simulink model "MdXX_RspToNetWork"  (R2024b)
settings: Solver=FixedStepDiscrete  StartTime=0.0  StopTime=10.0  FixedStep=0.01  RelTol=1e-3
(part 1 of 3)
settings Model: Creator=sn2xws  LastModifiedBy=sn55gm
settings Model: ModifiedHistory=|
  | 2024.8.20 v3.0.0 557增加Md53 Md56
  | 2024.10.15 V3.0.1 新增Md57 Md58
  | 25.7.8 V3.13.0 新增Md61 Md62
settings SolverCC: AlgebraicLoopSolver=TrustRegion
settings DataIOCC: SaveFormat=StructureWithTime  ReturnWorkspaceOutputs=off
settings OptimizationCC: DefaultParameterBehavior=Inlined  EnhancedBackFolding=on  PassReuseOutputArgsAs=Individual arguments  ZeroExternalMemoryAtStartup=off  ZeroInternalMemoryAtStartup=off  OptimizeBlockOrder=speed  DifferentSizesBufferReuse=on  OptimizationCustomize=off  EfficientTunableParamExpr=on
settings DebuggingCC: ParameterTunabilityLossMsg=error  UnconnectedInputMsg=warning  UnconnectedOutputMsg=warning  UnconnectedLineMsg=warning  ArithmeticOperatorsInVariantConditions=warning
settings ModelReferenceCC: EnableRefExpFcnMdlSchedulingChecks=on  ModelReferenceNumInstancesAllowed=Single
settings SFSimCC: MATLABDynamicMemAlloc=off  CustomCodeUndefinedFunction=UseInterfaceOnly
settings RTWCC: Description=AUTOSAR  SystemTargetFile=autosar.tlc  GenCodeOnly=on  TemplateMakefile=ert_default_tmf  GenerateReport=on  IncludeHyperlinkInReport=on  LaunchReport=on  DataTypeReplacement=CDataTypesFixedWidth  GenerateTraceInfo=on  GenerateTraceReport=on  GenerateTraceReportSl=on  GenerateTraceReportSf=on  GenerateTraceReportEml=on  GenerateCodeMetricsReport=on  GPUComputeCapability=3.5
settings CodeAppCC: ForceParamTrailComments=on  IgnoreCustomStorageClasses=off  OperatorAnnotations=on  SimulinkDataObjDesc=on  SFDataObjDesc=on  InsertBlockDesc=on
settings STFCustomTargetCC: TargetLangStandard=C99 (ISO)  MultiwordLength=256  ParMdlRefBuildCompliant=on  CompOptLevelCompliant=on  IncludeMdlTerminateFcn=off  CombineOutputUpdateFcns=on  SuppressErrorStatus=on  ERTCustomFileBanners=on  SupportNonFinite=off  SupportComplex=off  SupportContinuousTime=off  SupportNonInlinedSFcns=off  RemoveResetFunc=on  MATLABClassNameForMDSCustomization=Simulink.SoftwareTarget.ERTCustomization  AutosarCompliant=on  UseToolchainInfoCompliant=on  LookupTableObjectStructAxisOrder=2,1,3,4,...  LUTObjectStructOrderEvenSpacing=Size,Table,Breakpoints  SystemTargetFile=autosar.tlc
settings ERTTargetCC: TargetLangStandard=C99 (ISO)  ConcurrentExecutionCompliant=off  IncludeMdlTerminateFcn=off  SuppressErrorStatus=on  SupportNonFinite=off  SupportComplex=off  ModelStepFunctionPrototypeControlCompliant=off  CPPClassGenCompliant=off  AutosarCompliant=on  LookupTableObjectStructAxisOrder=2,1,3,4,...  LUTObjectStructOrderEvenSpacing=Size,Table,Breakpoints  ERTCustomFileTemplate=example_file_process.tlc  ERTFilePackagingFormat=Compact  BooleanTrueId=TRUE  BooleanFalseId=FALSE  DynamicArrayContainerType=coder::array

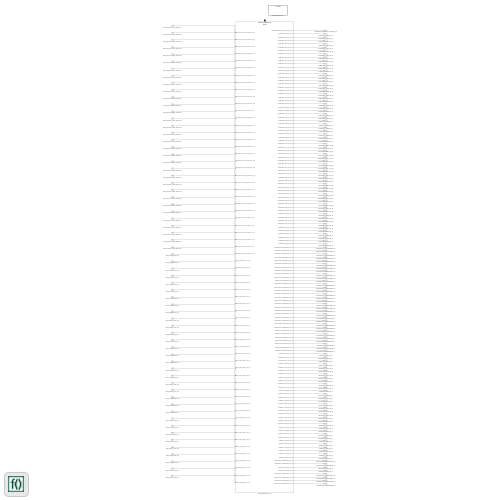
[thumbnail: Simulink's stored preview of the top-level diagram]
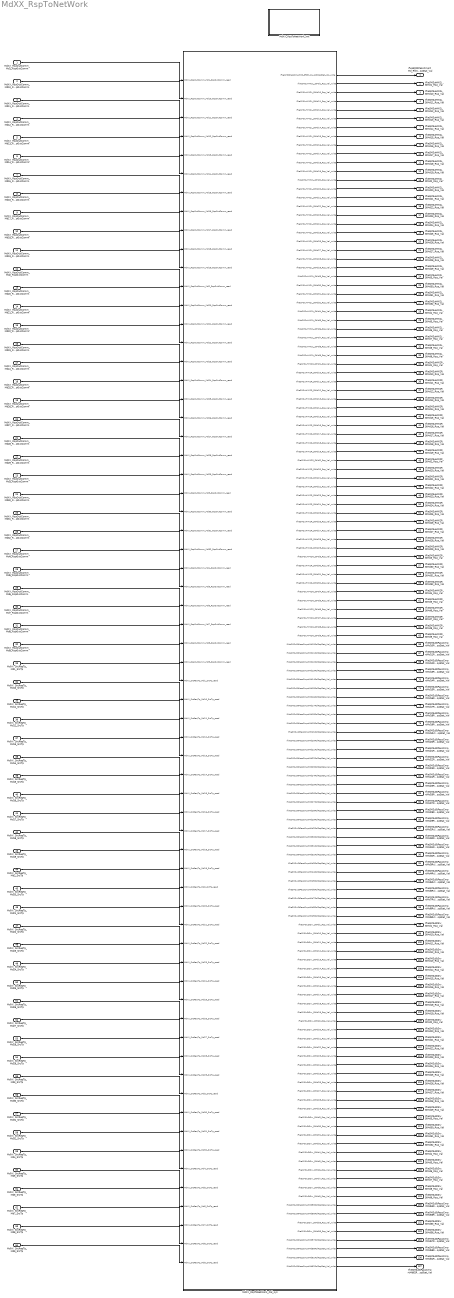
== system MdXX_RspToNetWork ==
  MdXX_RspOutComm_Md1_RspOutComm : Inport  OutDataTypeStr=uint8  PortDimensions=1
  MdXX_RspOutComm_Md10_RspOutComm : Inport  Port=2  OutDataTypeStr=uint8  PortDimensions=1
  MdXX_RspOutComm_Md11_RspOutComm : Inport  Port=3  OutDataTypeStr=uint8  PortDimensions=1
  MdXX_RspOutComm_Md12_RspOutComm : Inport  Port=4  OutDataTypeStr=uint8  PortDimensions=1
  MdXX_RspOutComm_Md13_RspOutComm : Inport  Port=5  OutDataTypeStr=uint8  PortDimensions=1
  MdXX_RspOutComm_Md14_RspOutComm : Inport  Port=6  OutDataTypeStr=uint8  PortDimensions=1
  MdXX_RspOutComm_Md15_RspOutComm : Inport  Port=7  OutDataTypeStr=uint8  PortDimensions=1
  MdXX_RspOutComm_Md16_RspOutComm : Inport  Port=8  OutDataTypeStr=uint8  PortDimensions=1
  MdXX_RspOutComm_Md17_RspOutComm : Inport  Port=9  OutDataTypeStr=uint8  PortDimensions=1
  MdXX_RspOutComm_Md18_RspOutComm : Inport  Port=10  OutDataTypeStr=uint8  PortDimensions=1
  MdXX_RspOutComm_Md19_RspOutComm : Inport  Port=11  OutDataTypeStr=uint8  PortDimensions=1
  MdXX_RspOutComm_Md2_RspOutComm : Inport  Port=12  OutDataTypeStr=uint8  PortDimensions=1
  MdXX_RspOutComm_Md20_RspOutComm : Inport  Port=13  OutDataTypeStr=uint8  PortDimensions=1
  MdXX_RspOutComm_Md21_RspOutComm : Inport  Port=14  OutDataTypeStr=uint8  PortDimensions=1
  MdXX_RspOutComm_Md22_RspOutComm : Inport  Port=15  OutDataTypeStr=uint8  PortDimensions=1
  MdXX_RspOutComm_Md23_RspOutComm : Inport  Port=16  OutDataTypeStr=uint8  PortDimensions=1
  MdXX_RspOutComm_Md24_RspOutComm : Inport  Port=17  OutDataTypeStr=uint8  PortDimensions=1
  MdXX_RspOutComm_Md25_RspOutComm : Inport  Port=18  OutDataTypeStr=uint8  PortDimensions=1
  MdXX_RspOutComm_Md26_RspOutComm : Inport  Port=19  OutDataTypeStr=uint8  PortDimensions=1
  MdXX_RspOutComm_Md27_RspOutComm : Inport  Port=20  OutDataTypeStr=uint8  PortDimensions=1
  MdXX_RspOutComm_Md28_RspOutComm : Inport  Port=21  OutDataTypeStr=uint8  PortDimensions=1
  MdXX_RspOutComm_Md29_RspOutComm : Inport  Port=22  OutDataTypeStr=uint8  PortDimensions=1
  MdXX_RspOutComm_Md3_RspOutComm : Inport  Port=23  OutDataTypeStr=uint8  PortDimensions=1
  MdXX_RspOutComm_Md30_RspOutComm : Inport  Port=24  OutDataTypeStr=uint8  PortDimensions=1
  MdXX_RspOutComm_Md31_RspOutComm : Inport  Port=25  OutDataTypeStr=uint8  PortDimensions=1
  MdXX_RspOutComm_Md32_RspOutComm : Inport  Port=26  OutDataTypeStr=uint8  PortDimensions=1
  MdXX_RspOutComm_Md4_RspOutComm : Inport  Port=27  OutDataTypeStr=uint8  PortDimensions=1
  MdXX_RspOutComm_Md5_RspOutComm : Inport  Port=28  OutDataTypeStr=uint8  PortDimensions=1
  MdXX_RspOutComm_Md6_RspOutComm : Inport  Port=29  OutDataTypeStr=uint8  PortDimensions=1
  MdXX_RspOutComm_Md7_RspOutComm : Inport  Port=30  OutDataTypeStr=uint8  PortDimensions=1
  MdXX_RspOutComm_Md8_RspOutComm : Inport  Port=31  OutDataTypeStr=uint8  PortDimensions=1
  MdXX_RspOutComm_Md9_RspOutComm : Inport  Port=32  OutDataTypeStr=uint8  PortDimensions=1
  MdXX_SrcReqTp_Md1_SrcTp : Inport  Port=33  OutDataTypeStr=Enum: SrcReqTp1  PortDimensions=1
  MdXX_SrcReqTp_Md10_SrcTp : Inport  Port=34  OutDataTypeStr=Enum: SrcReqTp1  PortDimensions=1
  MdXX_SrcReqTp_Md11_SrcTp : Inport  Port=35  OutDataTypeStr=Enum: SrcReqTp1  PortDimensions=1
  MdXX_SrcReqTp_Md12_SrcTp : Inport  Port=36  OutDataTypeStr=Enum: SrcReqTp1  PortDimensions=1
  MdXX_SrcReqTp_Md13_SrcTp : Inport  Port=37  OutDataTypeStr=Enum: SrcReqTp1  PortDimensions=1
  MdXX_SrcReqTp_Md14_SrcTp : Inport  Port=38  OutDataTypeStr=Enum: SrcReqTp1  PortDimensions=1
  MdXX_SrcReqTp_Md15_SrcTp : Inport  Port=39  OutDataTypeStr=Enum: SrcReqTp1  PortDimensions=1
  MdXX_SrcReqTp_Md16_SrcTp : Inport  Port=40  OutDataTypeStr=Enum: SrcReqTp1  PortDimensions=1
  MdXX_SrcReqTp_Md17_SrcTp : Inport  Port=41  OutDataTypeStr=Enum: SrcReqTp1  PortDimensions=1
  MdXX_SrcReqTp_Md18_SrcTp : Inport  Port=42  OutDataTypeStr=Enum: SrcReqTp1  PortDimensions=1
  MdXX_SrcReqTp_Md19_SrcTp : Inport  Port=43  OutDataTypeStr=Enum: SrcReqTp1  PortDimensions=1
  MdXX_SrcReqTp_Md2_SrcTp : Inport  Port=44  OutDataTypeStr=Enum: SrcReqTp1  PortDimensions=1
  MdXX_SrcReqTp_Md20_SrcTp : Inport  Port=45  OutDataTypeStr=Enum: SrcReqTp1  PortDimensions=1
  MdXX_SrcReqTp_Md21_SrcTp : Inport  Port=46  OutDataTypeStr=Enum: SrcReqTp1  PortDimensions=1
  MdXX_SrcReqTp_Md22_SrcTp : Inport  Port=47  OutDataTypeStr=Enum: SrcReqTp1  PortDimensions=1
  MdXX_SrcReqTp_Md23_SrcTp : Inport  Port=48  OutDataTypeStr=Enum: SrcReqTp1  PortDimensions=1
  MdXX_SrcReqTp_Md24_SrcTp : Inport  Port=49  OutDataTypeStr=Enum: SrcReqTp1  PortDimensions=1
  MdXX_SrcReqTp_Md25_SrcTp : Inport  Port=50  OutDataTypeStr=Enum: SrcReqTp1  PortDimensions=1
  MdXX_SrcReqTp_Md26_SrcTp : Inport  Port=51  OutDataTypeStr=Enum: SrcReqTp1  PortDimensions=1
  MdXX_SrcReqTp_Md27_SrcTp : Inport  Port=52  OutDataTypeStr=Enum: SrcReqTp1  PortDimensions=1
  MdXX_SrcReqTp_Md28_SrcTp : Inport  Port=53  OutDataTypeStr=Enum: SrcReqTp1  PortDimensions=1
  MdXX_SrcReqTp_Md29_SrcTp : Inport  Port=54  OutDataTypeStr=Enum: SrcReqTp1  PortDimensions=1
  MdXX_SrcReqTp_Md3_SrcTp : Inport  Port=55  OutDataTypeStr=Enum: SrcReqTp1  PortDimensions=1
  MdXX_SrcReqTp_Md30_SrcTp : Inport  Port=56  OutDataTypeStr=Enum: SrcReqTp1  PortDimensions=1
  MdXX_SrcReqTp_Md31_SrcTp : Inport  Port=57  OutDataTypeStr=Enum: SrcReqTp1  PortDimensions=1
  MdXX_SrcReqTp_Md32_SrcTp : Inport  Port=58  OutDataTypeStr=Enum: SrcReqTp1  PortDimensions=1
  MdXX_SrcReqTp_Md4_SrcTp : Inport  Port=59  OutDataTypeStr=Enum: SrcReqTp1  PortDimensions=1
  MdXX_SrcReqTp_Md5_SrcTp : Inport  Port=60  OutDataTypeStr=Enum: SrcReqTp1  PortDimensions=1
  MdXX_SrcReqTp_Md6_SrcTp : Inport  Port=61  OutDataTypeStr=Enum: SrcReqTp1  PortDimensions=1
  MdXX_SrcReqTp_Md7_SrcTp : Inport  Port=62  OutDataTypeStr=Enum: SrcReqTp1  PortDimensions=1
  MdXX_SrcReqTp_Md8_SrcTp : Inport  Port=63  OutDataTypeStr=Enum: SrcReqTp1  PortDimensions=1
  MdXX_SrcReqTp_Md9_SrcTp : Inport  Port=64  OutDataTypeStr=Enum: SrcReqTp1  PortDimensions=1
  MdXX_RspToNetWork_Cal_sys : Subsystem
  MdXX_RspToNetWork_Init : Subsystem
  IfVeSMStPassCmprtMd_RfCtrl_Sw_RclRspStat_Val : Outport  OutDataTypeStr=uint8  PortDimensions=1  VectorParamsAs1DForOutWhenUnconnected=off
  IfVeSMSuHMI2L_StMd1_Rsp_Val : Outport  Port=2  OutDataTypeStr=uint8  PortDimensions=1  VectorParamsAs1DForOutWhenUnconnected=off
  IfVeSMSuHMI2L_StMd10_Rsp_Val : Outport  Port=3  OutDataTypeStr=uint8  PortDimensions=1  VectorParamsAs1DForOutWhenUnconnected=off
  IfVeSMSuHMI2L_StMd11_Rsp_Val : Outport  Port=4  OutDataTypeStr=uint8  PortDimensions=1  VectorParamsAs1DForOutWhenUnconnected=off
  IfVeSMSuHMI2L_StMd12_Rsp_Val : Outport  Port=5  OutDataTypeStr=uint8  PortDimensions=1  VectorParamsAs1DForOutWhenUnconnected=off
  IfVeSMSuHMI2L_StMd13_Rsp_Val : Outport  Port=6  OutDataTypeStr=uint8  PortDimensions=1  VectorParamsAs1DForOutWhenUnconnected=off
  IfVeSMSuHMI2L_StMd14_Rsp_Val : Outport  Port=7  OutDataTypeStr=uint8  PortDimensions=1  VectorParamsAs1DForOutWhenUnconnected=off
  IfVeSMSuHMI2L_StMd15_Rsp_Val : Outport  Port=8  OutDataTypeStr=uint8  PortDimensions=1  VectorParamsAs1DForOutWhenUnconnected=off
  IfVeSMSuHMI2L_StMd16_Rsp_Val : Outport  Port=9  OutDataTypeStr=uint8  PortDimensions=1  VectorParamsAs1DForOutWhenUnconnected=off
  IfVeSMSuHMI2L_StMd17_Rsp_Val : Outport  Port=10  OutDataTypeStr=uint8  PortDimensions=1  VectorParamsAs1DForOutWhenUnconnected=off
  IfVeSMSuHMI2L_StMd18_Rsp_Val : Outport  Port=11  OutDataTypeStr=uint8  PortDimensions=1  VectorParamsAs1DForOutWhenUnconnected=off
  IfVeSMSuHMI2L_StMd19_Rsp_Val : Outport  Port=12  OutDataTypeStr=uint8  PortDimensions=1  VectorParamsAs1DForOutWhenUnconnected=off
  IfVeSMSuHMI2L_StMd2_Rsp_Val : Outport  Port=13  OutDataTypeStr=uint8  PortDimensions=1  VectorParamsAs1DForOutWhenUnconnected=off
  IfVeSMSuHMI2L_StMd20_Rsp_Val : Outport  Port=14  OutDataTypeStr=uint8  PortDimensions=1  VectorParamsAs1DForOutWhenUnconnected=off
  IfVeSMSuHMI2L_StMd21_Rsp_Val : Outport  Port=15  OutDataTypeStr=uint8  PortDimensions=1  VectorParamsAs1DForOutWhenUnconnected=off
  IfVeSMSuHMI2L_StMd22_Rsp_Val : Outport  Port=16  OutDataTypeStr=uint8  PortDimensions=1  VectorParamsAs1DForOutWhenUnconnected=off
  IfVeSMSuHMI2L_StMd23_Rsp_Val : Outport  Port=17  OutDataTypeStr=uint8  PortDimensions=1  VectorParamsAs1DForOutWhenUnconnected=off
  IfVeSMSuHMI2L_StMd24_Rsp_Val : Outport  Port=18  OutDataTypeStr=uint8  PortDimensions=1  VectorParamsAs1DForOutWhenUnconnected=off
  IfVeSMSuHMI2L_StMd25_Rsp_Val : Outport  Port=19  OutDataTypeStr=uint8  PortDimensions=1  VectorParamsAs1DForOutWhenUnconnected=off
  IfVeSMSuHMI2L_StMd26_Rsp_Val : Outport  Port=20  OutDataTypeStr=uint8  PortDimensions=1  VectorParamsAs1DForOutWhenUnconnected=off
  IfVeSMSuHMI2L_StMd27_Rsp_Val : Outport  Port=21  OutDataTypeStr=uint8  PortDimensions=1  VectorParamsAs1DForOutWhenUnconnected=off
  IfVeSMSuHMI2L_StMd28_Rsp_Val : Outport  Port=22  OutDataTypeStr=uint8  PortDimensions=1  VectorParamsAs1DForOutWhenUnconnected=off
  IfVeSMSuHMI2L_StMd29_Rsp_Val : Outport  Port=23  OutDataTypeStr=uint8  PortDimensions=1  VectorParamsAs1DForOutWhenUnconnected=off
  IfVeSMSuHMI2L_StMd3_Rsp_Val : Outport  Port=24  OutDataTypeStr=uint8  PortDimensions=1  VectorParamsAs1DForOutWhenUnconnected=off
  IfVeSMSuHMI2L_StMd30_Rsp_Val : Outport  Port=25  OutDataTypeStr=uint8  PortDimensions=1  VectorParamsAs1DForOutWhenUnconnected=off
  IfVeSMSuHMI2L_StMd31_Rsp_Val : Outport  Port=26  OutDataTypeStr=uint8  PortDimensions=1  VectorParamsAs1DForOutWhenUnconnected=off
  IfVeSMSuHMI2L_StMd32_Rsp_Val : Outport  Port=27  OutDataTypeStr=uint8  PortDimensions=1  VectorParamsAs1DForOutWhenUnconnected=off
  IfVeSMSuHMI2L_StMd4_Rsp_Val : Outport  Port=28  OutDataTypeStr=uint8  PortDimensions=1  VectorParamsAs1DForOutWhenUnconnected=off
  IfVeSMSuHMI2L_StMd5_Rsp_Val : Outport  Port=29  OutDataTypeStr=uint8  PortDimensions=1  VectorParamsAs1DForOutWhenUnconnected=off
  IfVeSMSuHMI2L_StMd6_Rsp_Val : Outport  Port=30  OutDataTypeStr=uint8  PortDimensions=1  VectorParamsAs1DForOutWhenUnconnected=off
  IfVeSMSuHMI2L_StMd7_Rsp_Val : Outport  Port=31  OutDataTypeStr=uint8  PortDimensions=1  VectorParamsAs1DForOutWhenUnconnected=off
  IfVeSMSuHMI2L_StMd8_Rsp_Val : Outport  Port=32  OutDataTypeStr=uint8  PortDimensions=1  VectorParamsAs1DForOutWhenUnconnected=off
  IfVeSMSuHMI2L_StMd9_Rsp_Val : Outport  Port=33  OutDataTypeStr=uint8  PortDimensions=1  VectorParamsAs1DForOutWhenUnconnected=off
  IfVeSMSuHMI2R_StMd1_Rsp_Val : Outport  Port=34  OutDataTypeStr=uint8  PortDimensions=1  VectorParamsAs1DForOutWhenUnconnected=off
  IfVeSMSuHMI2R_StMd10_Rsp_Val : Outport  Port=35  OutDataTypeStr=uint8  PortDimensions=1  VectorParamsAs1DForOutWhenUnconnected=off
  IfVeSMSuHMI2R_StMd11_Rsp_Val : Outport  Port=36  OutDataTypeStr=uint8  PortDimensions=1  VectorParamsAs1DForOutWhenUnconnected=off
  IfVeSMSuHMI2R_StMd12_Rsp_Val : Outport  Port=37  OutDataTypeStr=uint8  PortDimensions=1  VectorParamsAs1DForOutWhenUnconnected=off
  IfVeSMSuHMI2R_StMd13_Rsp_Val : Outport  Port=38  OutDataTypeStr=uint8  PortDimensions=1  VectorParamsAs1DForOutWhenUnconnected=off
  IfVeSMSuHMI2R_StMd14_Rsp_Val : Outport  Port=39  OutDataTypeStr=uint8  PortDimensions=1  VectorParamsAs1DForOutWhenUnconnected=off
  IfVeSMSuHMI2R_StMd15_Rsp_Val : Outport  Port=40  OutDataTypeStr=uint8  PortDimensions=1  VectorParamsAs1DForOutWhenUnconnected=off
  IfVeSMSuHMI2R_StMd16_Rsp_Val : Outport  Port=41  OutDataTypeStr=uint8  PortDimensions=1  VectorParamsAs1DForOutWhenUnconnected=off
  IfVeSMSuHMI2R_StMd17_Rsp_Val : Outport  Port=42  OutDataTypeStr=uint8  PortDimensions=1  VectorParamsAs1DForOutWhenUnconnected=off
  IfVeSMSuHMI2R_StMd18_Rsp_Val : Outport  Port=43  OutDataTypeStr=uint8  PortDimensions=1  VectorParamsAs1DForOutWhenUnconnected=off
  IfVeSMSuHMI2R_StMd19_Rsp_Val : Outport  Port=44  OutDataTypeStr=uint8  PortDimensions=1  VectorParamsAs1DForOutWhenUnconnected=off
  IfVeSMSuHMI2R_StMd2_Rsp_Val : Outport  Port=45  OutDataTypeStr=uint8  PortDimensions=1  VectorParamsAs1DForOutWhenUnconnected=off
  IfVeSMSuHMI2R_StMd20_Rsp_Val : Outport  Port=46  OutDataTypeStr=uint8  PortDimensions=1  VectorParamsAs1DForOutWhenUnconnected=off
  IfVeSMSuHMI2R_StMd21_Rsp_Val : Outport  Port=47  OutDataTypeStr=uint8  PortDimensions=1  VectorParamsAs1DForOutWhenUnconnected=off
  IfVeSMSuHMI2R_StMd22_Rsp_Val : Outport  Port=48  OutDataTypeStr=uint8  PortDimensions=1  VectorParamsAs1DForOutWhenUnconnected=off
  IfVeSMSuHMI2R_StMd23_Rsp_Val : Outport  Port=49  OutDataTypeStr=uint8  PortDimensions=1  VectorParamsAs1DForOutWhenUnconnected=off
  IfVeSMSuHMI2R_StMd24_Rsp_Val : Outport  Port=50  OutDataTypeStr=uint8  PortDimensions=1  VectorParamsAs1DForOutWhenUnconnected=off
  IfVeSMSuHMI2R_StMd25_Rsp_Val : Outport  Port=51  OutDataTypeStr=uint8  PortDimensions=1  VectorParamsAs1DForOutWhenUnconnected=off
  IfVeSMSuHMI2R_StMd26_Rsp_Val : Outport  Port=52  OutDataTypeStr=uint8  PortDimensions=1  VectorParamsAs1DForOutWhenUnconnected=off
  IfVeSMSuHMI2R_StMd27_Rsp_Val : Outport  Port=53  OutDataTypeStr=uint8  PortDimensions=1  VectorParamsAs1DForOutWhenUnconnected=off
  IfVeSMSuHMI2R_StMd28_Rsp_Val : Outport  Port=54  OutDataTypeStr=uint8  PortDimensions=1  VectorParamsAs1DForOutWhenUnconnected=off
  IfVeSMSuHMI2R_StMd29_Rsp_Val : Outport  Port=55  OutDataTypeStr=uint8  PortDimensions=1  VectorParamsAs1DForOutWhenUnconnected=off
  IfVeSMSuHMI2R_StMd3_Rsp_Val : Outport  Port=56  OutDataTypeStr=uint8  PortDimensions=1  VectorParamsAs1DForOutWhenUnconnected=off
  IfVeSMSuHMI2R_StMd30_Rsp_Val : Outport  Port=57  OutDataTypeStr=uint8  PortDimensions=1  VectorParamsAs1DForOutWhenUnconnected=off
  IfVeSMSuHMI2R_StMd31_Rsp_Val : Outport  Port=58  OutDataTypeStr=uint8  PortDimensions=1  VectorParamsAs1DForOutWhenUnconnected=off
  IfVeSMSuHMI2R_StMd32_Rsp_Val : Outport  Port=59  OutDataTypeStr=uint8  PortDimensions=1  VectorParamsAs1DForOutWhenUnconnected=off
  IfVeSMSuHMI2R_StMd4_Rsp_Val : Outport  Port=60  OutDataTypeStr=uint8  PortDimensions=1  VectorParamsAs1DForOutWhenUnconnected=off
  IfVeSMSuHMI2R_StMd5_Rsp_Val : Outport  Port=61  OutDataTypeStr=uint8  PortDimensions=1  VectorParamsAs1DForOutWhenUnconnected=off
  IfVeSMSuHMI2R_StMd6_Rsp_Val : Outport  Port=62  OutDataTypeStr=uint8  PortDimensions=1  VectorParamsAs1DForOutWhenUnconnected=off
  IfVeSMSuHMI2R_StMd7_Rsp_Val : Outport  Port=63  OutDataTypeStr=uint8  PortDimensions=1  VectorParamsAs1DForOutWhenUnconnected=off
  IfVeSMSuHMI2R_StMd8_Rsp_Val : Outport  Port=64  OutDataTypeStr=uint8  PortDimensions=1  VectorParamsAs1DForOutWhenUnconnected=off
  IfVeSMSuHMI2R_StMd9_Rsp_Val : Outport  Port=65  OutDataTypeStr=uint8  PortDimensions=1  VectorParamsAs1DForOutWhenUnconnected=off
  IfVeSMSuStPassCmprtMd10RclRspStat_Val : Outport  Port=66  OutDataTypeStr=uint8  PortDimensions=1  VectorParamsAs1DForOutWhenUnconnected=off
  IfVeSMSuStPassCmprtMd11RclRspStat_Val : Outport  Port=67  OutDataTypeStr=uint8  PortDimensions=1  VectorParamsAs1DForOutWhenUnconnected=off
  IfVeSMSuStPassCmprtMd12RclRspStat_Val : Outport  Port=68  OutDataTypeStr=uint8  PortDimensions=1  VectorParamsAs1DForOutWhenUnconnected=off
  IfVeSMSuStPassCmprtMd13RclRspStat_Val : Outport  Port=69  OutDataTypeStr=uint8  PortDimensions=1  VectorParamsAs1DForOutWhenUnconnected=off
  IfVeSMSuStPassCmprtMd14RclRspStat_Val : Outport  Port=70  OutDataTypeStr=uint8  PortDimensions=1  VectorParamsAs1DForOutWhenUnconnected=off
  IfVeSMSuStPassCmprtMd15RclRspStat_Val : Outport  Port=71  OutDataTypeStr=uint8  PortDimensions=1  VectorParamsAs1DForOutWhenUnconnected=off
  IfVeSMSuStPassCmprtMd16RclRspStat_Val : Outport  Port=72  OutDataTypeStr=uint8  PortDimensions=1  VectorParamsAs1DForOutWhenUnconnected=off
  IfVeSMSuStPassCmprtMd17RclRspStat_Val : Outport  Port=73  OutDataTypeStr=uint8  PortDimensions=1  VectorParamsAs1DForOutWhenUnconnected=off
  IfVeSMSuStPassCmprtMd18RclRspStat_Val : Outport  Port=74  OutDataTypeStr=uint8  PortDimensions=1  VectorParamsAs1DForOutWhenUnconnected=off
  IfVeSMSuStPassCmprtMd19RclRspStat_Val : Outport  Port=75  OutDataTypeStr=uint8  PortDimensions=1  VectorParamsAs1DForOutWhenUnconnected=off
  IfVeSMSuStPassCmprtMd1RclRspStat_Val : Outport  Port=76  OutDataTypeStr=uint8  PortDimensions=1  VectorParamsAs1DForOutWhenUnconnected=off
  IfVeSMSuStPassCmprtMd20RclRspStat_Val : Outport  Port=77  OutDataTypeStr=uint8  PortDimensions=1  VectorParamsAs1DForOutWhenUnconnected=off
  IfVeSMSuStPassCmprtMd21RclRspStat_Val : Outport  Port=78  OutDataTypeStr=uint8  PortDimensions=1  VectorParamsAs1DForOutWhenUnconnected=off
  IfVeSMSuStPassCmprtMd22RclRspStat_Val : Outport  Port=79  OutDataTypeStr=uint8  PortDimensions=1  VectorParamsAs1DForOutWhenUnconnected=off
  IfVeSMSuStPassCmprtMd23RclRspStat_Val : Outport  Port=80  OutDataTypeStr=uint8  PortDimensions=1  VectorParamsAs1DForOutWhenUnconnected=off
  IfVeSMSuStPassCmprtMd24RclRspStat_Val : Outport  Port=81  OutDataTypeStr=uint8  PortDimensions=1  VectorParamsAs1DForOutWhenUnconnected=off
  IfVeSMSuStPassCmprtMd25RclRspStat_Val : Outport  Port=82  OutDataTypeStr=uint8  PortDimensions=1  VectorParamsAs1DForOutWhenUnconnected=off
  IfVeSMSuStPassCmprtMd26RclRspStat_Val : Outport  Port=83  OutDataTypeStr=uint8  PortDimensions=1  VectorParamsAs1DForOutWhenUnconnected=off
  IfVeSMSuStPassCmprtMd27RclRspStat_Val : Outport  Port=84  OutDataTypeStr=uint8  PortDimensions=1  VectorParamsAs1DForOutWhenUnconnected=off
  IfVeSMSuStPassCmprtMd28RclRspStat_Val : Outport  Port=85  OutDataTypeStr=uint8  PortDimensions=1  VectorParamsAs1DForOutWhenUnconnected=off
  IfVeSMSuStPassCmprtMd29RclRspStat_Val : Outport  Port=86  OutDataTypeStr=uint8  PortDimensions=1  VectorParamsAs1DForOutWhenUnconnected=off
  IfVeSMSuStPassCmprtMd2RclRspStat_Val : Outport  Port=87  OutDataTypeStr=uint8  PortDimensions=1  VectorParamsAs1DForOutWhenUnconnected=off
  IfVeSMSuStPassCmprtMd30RclRspStat_Val : Outport  Port=88  OutDataTypeStr=uint8  PortDimensions=1  VectorParamsAs1DForOutWhenUnconnected=off
  IfVeSMSuStPassCmprtMd31RclRspStat_Val : Outport  Port=89  OutDataTypeStr=uint8  PortDimensions=1  VectorParamsAs1DForOutWhenUnconnected=off
  IfVeSMSuStPassCmprtMd32RclRspStat_Val : Outport  Port=90  OutDataTypeStr=uint8  PortDimensions=1  VectorParamsAs1DForOutWhenUnconnected=off
  IfVeSMSuStPassCmprtMd3RclRspStat_Val : Outport  Port=91  OutDataTypeStr=uint8  PortDimensions=1  VectorParamsAs1DForOutWhenUnconnected=off
  IfVeSMSuStPassCmprtMd4RclRspStat_Val : Outport  Port=92  OutDataTypeStr=uint8  PortDimensions=1  VectorParamsAs1DForOutWhenUnconnected=off
  IfVeSMSuStPassCmprtMd5RclRspStat_Val : Outport  Port=93  OutDataTypeStr=uint8  PortDimensions=1  VectorParamsAs1DForOutWhenUnconnected=off
  IfVeSMSuStPassCmprtMd6RclRspStat_Val : Outport  Port=94  OutDataTypeStr=uint8  PortDimensions=1  VectorParamsAs1DForOutWhenUnconnected=off
  IfVeSMSuStPassCmprtMd7RclRspStat_Val : Outport  Port=95  OutDataTypeStr=uint8  PortDimensions=1  VectorParamsAs1DForOutWhenUnconnected=off
  IfVeSMSuStPassCmprtMd8RclRspStat_Val : Outport  Port=96  OutDataTypeStr=uint8  PortDimensions=1  VectorParamsAs1DForOutWhenUnconnected=off
  IfVeSMSuStPassCmprtMd9RclRspStat_Val : Outport  Port=97  OutDataTypeStr=uint8  PortDimensions=1  VectorParamsAs1DForOutWhenUnconnected=off
  IfVeSMSuStSrv_StMd1_Rsp_Val : Outport  Port=98  OutDataTypeStr=uint8  PortDimensions=1  VectorParamsAs1DForOutWhenUnconnected=off
  IfVeSMSuStSrv_StMd10_Rsp_Val : Outport  Port=99  OutDataTypeStr=uint8  PortDimensions=1  VectorParamsAs1DForOutWhenUnconnected=off
  IfVeSMSuStSrv_StMd11_Rsp_Val : Outport  Port=100  OutDataTypeStr=uint8  PortDimensions=1  VectorParamsAs1DForOutWhenUnconnected=off
  IfVeSMSuStSrv_StMd12_Rsp_Val : Outport  Port=101  OutDataTypeStr=uint8  PortDimensions=1  VectorParamsAs1DForOutWhenUnconnected=off
  IfVeSMSuStSrv_StMd13_Rsp_Val : Outport  Port=102  OutDataTypeStr=uint8  PortDimensions=1  VectorParamsAs1DForOutWhenUnconnected=off
  IfVeSMSuStSrv_StMd14_Rsp_Val : Outport  Port=103  OutDataTypeStr=uint8  PortDimensions=1  VectorParamsAs1DForOutWhenUnconnected=off
  IfVeSMSuStSrv_StMd15_Rsp_Val : Outport  Port=104  OutDataTypeStr=uint8  PortDimensions=1  VectorParamsAs1DForOutWhenUnconnected=off
  IfVeSMSuStSrv_StMd16_Rsp_Val : Outport  Port=105  OutDataTypeStr=uint8  PortDimensions=1  VectorParamsAs1DForOutWhenUnconnected=off
  IfVeSMSuStSrv_StMd17_Rsp_Val : Outport  Port=106  OutDataTypeStr=uint8  PortDimensions=1  VectorParamsAs1DForOutWhenUnconnected=off
  IfVeSMSuStSrv_StMd18_Rsp_Val : Outport  Port=107  OutDataTypeStr=uint8  PortDimensions=1  VectorParamsAs1DForOutWhenUnconnected=off
  IfVeSMSuStSrv_StMd19_Rsp_Val : Outport  Port=108  OutDataTypeStr=uint8  PortDimensions=1  VectorParamsAs1DForOutWhenUnconnected=off
  IfVeSMSuStSrv_StMd2_Rsp_Val : Outport  Port=109  OutDataTypeStr=uint8  PortDimensions=1  VectorParamsAs1DForOutWhenUnconnected=off
  IfVeSMSuStSrv_StMd20_Rsp_Val : Outport  Port=110  OutDataTypeStr=uint8  PortDimensions=1  VectorParamsAs1DForOutWhenUnconnected=off
  IfVeSMSuStSrv_StMd21_Rsp_Val : Outport  Port=111  OutDataTypeStr=uint8  PortDimensions=1  VectorParamsAs1DForOutWhenUnconnected=off
  IfVeSMSuStSrv_StMd22_Rsp_Val : Outport  Port=112  OutDataTypeStr=uint8  PortDimensions=1  VectorParamsAs1DForOutWhenUnconnected=off
  IfVeSMSuStSrv_StMd23_Rsp_Val : Outport  Port=113  OutDataTypeStr=uint8  PortDimensions=1  VectorParamsAs1DForOutWhenUnconnected=off
  IfVeSMSuStSrv_StMd24_Rsp_Val : Outport  Port=114  OutDataTypeStr=uint8  PortDimensions=1  VectorParamsAs1DForOutWhenUnconnected=off
  IfVeSMSuStSrv_StMd25_Rsp_Val : Outport  Port=115  OutDataTypeStr=uint8  PortDimensions=1  VectorParamsAs1DForOutWhenUnconnected=off
  IfVeSMSuStSrv_StMd26_Rsp_Val : Outport  Port=116  OutDataTypeStr=uint8  PortDimensions=1  VectorParamsAs1DForOutWhenUnconnected=off
  IfVeSMSuStSrv_StMd27_Rsp_Val : Outport  Port=117  OutDataTypeStr=uint8  PortDimensions=1  VectorParamsAs1DForOutWhenUnconnected=off
  IfVeSMSuStSrv_StMd28_Rsp_Val : Outport  Port=118  OutDataTypeStr=uint8  PortDimensions=1  VectorParamsAs1DForOutWhenUnconnected=off
  IfVeSMSuStSrv_StMd29_Rsp_Val : Outport  Port=119  OutDataTypeStr=uint8  PortDimensions=1  VectorParamsAs1DForOutWhenUnconnected=off
  IfVeSMSuStSrv_StMd3_Rsp_Val : Outport  Port=120  OutDataTypeStr=uint8  PortDimensions=1  VectorParamsAs1DForOutWhenUnconnected=off
  IfVeSMSuStSrv_StMd30_Rsp_Val : Outport  Port=121  OutDataTypeStr=uint8  PortDimensions=1  VectorParamsAs1DForOutWhenUnconnected=off
  IfVeSMSuStSrv_StMd31_Rsp_Val : Outport  Port=122  OutDataTypeStr=uint8  PortDimensions=1  VectorParamsAs1DForOutWhenUnconnected=off
  IfVeSMSuStSrv_StMd32_Rsp_Val : Outport  Port=123  OutDataTypeStr=uint8  PortDimensions=1  VectorParamsAs1DForOutWhenUnconnected=off
  IfVeSMSuStSrv_StMd4_Rsp_Val : Outport  Port=124  OutDataTypeStr=uint8  PortDimensions=1  VectorParamsAs1DForOutWhenUnconnected=off
  IfVeSMSuStSrv_StMd5_Rsp_Val : Outport  Port=125  OutDataTypeStr=uint8  PortDimensions=1  VectorParamsAs1DForOutWhenUnconnected=off
  IfVeSMSuStSrv_StMd6_Rsp_Val : Outport  Port=126  OutDataTypeStr=uint8  PortDimensions=1  VectorParamsAs1DForOutWhenUnconnected=off
  IfVeSMSuStSrv_StMd7_Rsp_Val : Outport  Port=127  OutDataTypeStr=uint8  PortDimensions=1  VectorParamsAs1DForOutWhenUnconnected=off
  IfVeSMSuStSrv_StMd8_Rsp_Val : Outport  Port=128  OutDataTypeStr=uint8  PortDimensions=1  VectorParamsAs1DForOutWhenUnconnected=off
  IfVeSMSuStSrv_StMd9_Rsp_Val : Outport  Port=129  OutDataTypeStr=uint8  PortDimensions=1  VectorParamsAs1DForOutWhenUnconnected=off
  IfVeSMSuStPassCmprtMd53RclRspStat_Val : Outport  Port=130  OutDataTypeStr=uint8  PortDimensions=1  VectorParamsAs1DForOutWhenUnconnected=off
  IfVeSMSuStPassCmprtMd56RclRspStat_Val : Outport  Port=131  OutDataTypeStr=uint8  PortDimensions=1  VectorParamsAs1DForOutWhenUnconnected=off
  IfVeSMSuStSrv_StMd53_Rsp_Val : Outport  Port=132  OutDataTypeStr=uint8  PortDimensions=1  VectorParamsAs1DForOutWhenUnconnected=off
  IfVeSMSuStSrv_StMd56_Rsp_Val : Outport  Port=133  OutDataTypeStr=uint8  PortDimensions=1  VectorParamsAs1DForOutWhenUnconnected=off
  IfVeSMSuStPassCmprtMd57RclRspStat_Val : Outport  Port=134  OutDataTypeStr=uint8  PortDimensions=1  VectorParamsAs1DForOutWhenUnconnected=off
  IfVeSMSuStPassCmprtMd58RclRspStat_Val : Outport  Port=135  OutDataTypeStr=uint8  PortDimensions=1  VectorParamsAs1DForOutWhenUnconnected=off
  IfVeSMSuStPassCmprtMd61RclRspStat_Val : Outport  Port=136  OutDataTypeStr=uint8  PortDimensions=1  VectorParamsAs1DForOutWhenUnconnected=off
  IfVeSMSuStPassCmprtMd62RclRspStat_Val : Outport  Port=137  OutDataTypeStr=uint8  PortDimensions=1  VectorParamsAs1DForOutWhenUnconnected=off
  wires:
  MdXX_RspOutComm_Md1_RspOutComm/1 -> MdXX_RspToNetWork_Cal_sys/1(MdXX_RspOutComm_Md1_RspOutComm_read)
  MdXX_RspOutComm_Md10_RspOutComm/1 -> MdXX_RspToNetWork_Cal_sys/2(MdXX_RspOutComm_Md10_RspOutComm_read)
  MdXX_RspOutComm_Md11_RspOutComm/1 -> MdXX_RspToNetWork_Cal_sys/3(MdXX_RspOutComm_Md11_RspOutComm_read)
  MdXX_RspOutComm_Md12_RspOutComm/1 -> MdXX_RspToNetWork_Cal_sys/4(MdXX_RspOutComm_Md12_RspOutComm_read)
  MdXX_RspOutComm_Md13_RspOutComm/1 -> MdXX_RspToNetWork_Cal_sys/5(MdXX_RspOutComm_Md13_RspOutComm_read)
  MdXX_RspOutComm_Md14_RspOutComm/1 -> MdXX_RspToNetWork_Cal_sys/6(MdXX_RspOutComm_Md14_RspOutComm_read)
  MdXX_RspOutComm_Md15_RspOutComm/1 -> MdXX_RspToNetWork_Cal_sys/7(MdXX_RspOutComm_Md15_RspOutComm_read)
  MdXX_RspOutComm_Md16_RspOutComm/1 -> MdXX_RspToNetWork_Cal_sys/8(MdXX_RspOutComm_Md16_RspOutComm_read)
  MdXX_RspOutComm_Md17_RspOutComm/1 -> MdXX_RspToNetWork_Cal_sys/9(MdXX_RspOutComm_Md17_RspOutComm_read)
  MdXX_RspOutComm_Md18_RspOutComm/1 -> MdXX_RspToNetWork_Cal_sys/10(MdXX_RspOutComm_Md18_RspOutComm_read)
  MdXX_RspOutComm_Md19_RspOutComm/1 -> MdXX_RspToNetWork_Cal_sys/11(MdXX_RspOutComm_Md19_RspOutComm_read)
  MdXX_RspOutComm_Md2_RspOutComm/1 -> MdXX_RspToNetWork_Cal_sys/12(MdXX_RspOutComm_Md2_RspOutComm_read)
  MdXX_RspOutComm_Md20_RspOutComm/1 -> MdXX_RspToNetWork_Cal_sys/13(MdXX_RspOutComm_Md20_RspOutComm_read)
  MdXX_RspOutComm_Md21_RspOutComm/1 -> MdXX_RspToNetWork_Cal_sys/14(MdXX_RspOutComm_Md21_RspOutComm_read)
  MdXX_RspOutComm_Md22_RspOutComm/1 -> MdXX_RspToNetWork_Cal_sys/15(MdXX_RspOutComm_Md22_RspOutComm_read)
  MdXX_RspOutComm_Md23_RspOutComm/1 -> MdXX_RspToNetWork_Cal_sys/16(MdXX_RspOutComm_Md23_RspOutComm_read)
  MdXX_RspOutComm_Md24_RspOutComm/1 -> MdXX_RspToNetWork_Cal_sys/17(MdXX_RspOutComm_Md24_RspOutComm_read)
  MdXX_RspOutComm_Md25_RspOutComm/1 -> MdXX_RspToNetWork_Cal_sys/18(MdXX_RspOutComm_Md25_RspOutComm_read)
  MdXX_RspOutComm_Md26_RspOutComm/1 -> MdXX_RspToNetWork_Cal_sys/19(MdXX_RspOutComm_Md26_RspOutComm_read)
  MdXX_RspOutComm_Md27_RspOutComm/1 -> MdXX_RspToNetWork_Cal_sys/20(MdXX_RspOutComm_Md27_RspOutComm_read)
  MdXX_RspOutComm_Md28_RspOutComm/1 -> MdXX_RspToNetWork_Cal_sys/21(MdXX_RspOutComm_Md28_RspOutComm_read)
  MdXX_RspOutComm_Md29_RspOutComm/1 -> MdXX_RspToNetWork_Cal_sys/22(MdXX_RspOutComm_Md29_RspOutComm_read)
  MdXX_RspOutComm_Md3_RspOutComm/1 -> MdXX_RspToNetWork_Cal_sys/23(MdXX_RspOutComm_Md3_RspOutComm_read)
  MdXX_RspOutComm_Md30_RspOutComm/1 -> MdXX_RspToNetWork_Cal_sys/24(MdXX_RspOutComm_Md30_RspOutComm_read)
  MdXX_RspOutComm_Md31_RspOutComm/1 -> MdXX_RspToNetWork_Cal_sys/25(MdXX_RspOutComm_Md31_RspOutComm_read)
  MdXX_RspOutComm_Md32_RspOutComm/1 -> MdXX_RspToNetWork_Cal_sys/26(MdXX_RspOutComm_Md32_RspOutComm_read)
  MdXX_RspOutComm_Md4_RspOutComm/1 -> MdXX_RspToNetWork_Cal_sys/27(MdXX_RspOutComm_Md4_RspOutComm_read)
  MdXX_RspOutComm_Md5_RspOutComm/1 -> MdXX_RspToNetWork_Cal_sys/28(MdXX_RspOutComm_Md5_RspOutComm_read)
  MdXX_RspOutComm_Md6_RspOutComm/1 -> MdXX_RspToNetWork_Cal_sys/29(MdXX_RspOutComm_Md6_RspOutComm_read)
  MdXX_RspOutComm_Md7_RspOutComm/1 -> MdXX_RspToNetWork_Cal_sys/30(MdXX_RspOutComm_Md7_RspOutComm_read)
  MdXX_RspOutComm_Md8_RspOutComm/1 -> MdXX_RspToNetWork_Cal_sys/31(MdXX_RspOutComm_Md8_RspOutComm_read)
  MdXX_RspOutComm_Md9_RspOutComm/1 -> MdXX_RspToNetWork_Cal_sys/32(MdXX_RspOutComm_Md9_RspOutComm_read)
  MdXX_SrcReqTp_Md1_SrcTp/1 -> MdXX_RspToNetWork_Cal_sys/33(MdXX_SrcReqTp_Md1_SrcTp_read)
  MdXX_SrcReqTp_Md10_SrcTp/1 -> MdXX_RspToNetWork_Cal_sys/34(MdXX_SrcReqTp_Md10_SrcTp_read)
  MdXX_SrcReqTp_Md11_SrcTp/1 -> MdXX_RspToNetWork_Cal_sys/35(MdXX_SrcReqTp_Md11_SrcTp_read)
  MdXX_SrcReqTp_Md12_SrcTp/1 -> MdXX_RspToNetWork_Cal_sys/36(MdXX_SrcReqTp_Md12_SrcTp_read)
  MdXX_SrcReqTp_Md13_SrcTp/1 -> MdXX_RspToNetWork_Cal_sys/37(MdXX_SrcReqTp_Md13_SrcTp_read)
  MdXX_SrcReqTp_Md14_SrcTp/1 -> MdXX_RspToNetWork_Cal_sys/38(MdXX_SrcReqTp_Md14_SrcTp_read)
  MdXX_SrcReqTp_Md15_SrcTp/1 -> MdXX_RspToNetWork_Cal_sys/39(MdXX_SrcReqTp_Md15_SrcTp_read)
  MdXX_SrcReqTp_Md16_SrcTp/1 -> MdXX_RspToNetWork_Cal_sys/40(MdXX_SrcReqTp_Md16_SrcTp_read)
  MdXX_SrcReqTp_Md17_SrcTp/1 -> MdXX_RspToNetWork_Cal_sys/41(MdXX_SrcReqTp_Md17_SrcTp_read)
  MdXX_SrcReqTp_Md18_SrcTp/1 -> MdXX_RspToNetWork_Cal_sys/42(MdXX_SrcReqTp_Md18_SrcTp_read)
  MdXX_SrcReqTp_Md19_SrcTp/1 -> MdXX_RspToNetWork_Cal_sys/43(MdXX_SrcReqTp_Md19_SrcTp_read)
  MdXX_SrcReqTp_Md2_SrcTp/1 -> MdXX_RspToNetWork_Cal_sys/44(MdXX_SrcReqTp_Md2_SrcTp_read)
  MdXX_SrcReqTp_Md20_SrcTp/1 -> MdXX_RspToNetWork_Cal_sys/45(MdXX_SrcReqTp_Md20_SrcTp_read)
  MdXX_SrcReqTp_Md21_SrcTp/1 -> MdXX_RspToNetWork_Cal_sys/46(MdXX_SrcReqTp_Md21_SrcTp_read)
  MdXX_SrcReqTp_Md22_SrcTp/1 -> MdXX_RspToNetWork_Cal_sys/47(MdXX_SrcReqTp_Md22_SrcTp_read)
  MdXX_SrcReqTp_Md23_SrcTp/1 -> MdXX_RspToNetWork_Cal_sys/48(MdXX_SrcReqTp_Md23_SrcTp_read)
  MdXX_SrcReqTp_Md24_SrcTp/1 -> MdXX_RspToNetWork_Cal_sys/49(MdXX_SrcReqTp_Md24_SrcTp_read)
  MdXX_SrcReqTp_Md25_SrcTp/1 -> MdXX_RspToNetWork_Cal_sys/50(MdXX_SrcReqTp_Md25_SrcTp_read)
  MdXX_SrcReqTp_Md26_SrcTp/1 -> MdXX_RspToNetWork_Cal_sys/51(MdXX_SrcReqTp_Md26_SrcTp_read)
  MdXX_SrcReqTp_Md27_SrcTp/1 -> MdXX_RspToNetWork_Cal_sys/52(MdXX_SrcReqTp_Md27_SrcTp_read)
  MdXX_SrcReqTp_Md28_SrcTp/1 -> MdXX_RspToNetWork_Cal_sys/53(MdXX_SrcReqTp_Md28_SrcTp_read)
  MdXX_SrcReqTp_Md29_SrcTp/1 -> MdXX_RspToNetWork_Cal_sys/54(MdXX_SrcReqTp_Md29_SrcTp_read)
  MdXX_SrcReqTp_Md3_SrcTp/1 -> MdXX_RspToNetWork_Cal_sys/55(MdXX_SrcReqTp_Md3_SrcTp_read)
  MdXX_SrcReqTp_Md30_SrcTp/1 -> MdXX_RspToNetWork_Cal_sys/56(MdXX_SrcReqTp_Md30_SrcTp_read)
  MdXX_SrcReqTp_Md31_SrcTp/1 -> MdXX_RspToNetWork_Cal_sys/57(MdXX_SrcReqTp_Md31_SrcTp_read)
  MdXX_SrcReqTp_Md32_SrcTp/1 -> MdXX_RspToNetWork_Cal_sys/58(MdXX_SrcReqTp_Md32_SrcTp_read)
  MdXX_SrcReqTp_Md4_SrcTp/1 -> MdXX_RspToNetWork_Cal_sys/59(MdXX_SrcReqTp_Md4_SrcTp_read)
  MdXX_SrcReqTp_Md5_SrcTp/1 -> MdXX_RspToNetWork_Cal_sys/60(MdXX_SrcReqTp_Md5_SrcTp_read)
  MdXX_SrcReqTp_Md6_SrcTp/1 -> MdXX_RspToNetWork_Cal_sys/61(MdXX_SrcReqTp_Md6_SrcTp_read)
  MdXX_SrcReqTp_Md7_SrcTp/1 -> MdXX_RspToNetWork_Cal_sys/62(MdXX_SrcReqTp_Md7_SrcTp_read)
  MdXX_SrcReqTp_Md8_SrcTp/1 -> MdXX_RspToNetWork_Cal_sys/63(MdXX_SrcReqTp_Md8_SrcTp_read)
  MdXX_SrcReqTp_Md9_SrcTp/1 -> MdXX_RspToNetWork_Cal_sys/64(MdXX_SrcReqTp_Md9_SrcTp_read)
  MdXX_RspToNetWork_Cal_sys/1(IfVeSMStPassCmprtMd_RfCtrl_Sw_RclRspStat_Val_write) -> IfVeSMStPassCmprtMd_RfCtrl_Sw_RclRspStat_Val/1
  MdXX_RspToNetWork_Cal_sys/2(IfVeSMSuHMI2L_StMd1_Rsp_Val_write) -> IfVeSMSuHMI2L_StMd1_Rsp_Val/1
  MdXX_RspToNetWork_Cal_sys/3(IfVeSMSuHMI2L_StMd10_Rsp_Val_write) -> IfVeSMSuHMI2L_StMd10_Rsp_Val/1
  MdXX_RspToNetWork_Cal_sys/4(IfVeSMSuHMI2L_StMd11_Rsp_Val_write) -> IfVeSMSuHMI2L_StMd11_Rsp_Val/1
  MdXX_RspToNetWork_Cal_sys/5(IfVeSMSuHMI2L_StMd12_Rsp_Val_write) -> IfVeSMSuHMI2L_StMd12_Rsp_Val/1
  MdXX_RspToNetWork_Cal_sys/6(IfVeSMSuHMI2L_StMd13_Rsp_Val_write) -> IfVeSMSuHMI2L_StMd13_Rsp_Val/1
  MdXX_RspToNetWork_Cal_sys/7(IfVeSMSuHMI2L_StMd14_Rsp_Val_write) -> IfVeSMSuHMI2L_StMd14_Rsp_Val/1
  MdXX_RspToNetWork_Cal_sys/8(IfVeSMSuHMI2L_StMd15_Rsp_Val_write) -> IfVeSMSuHMI2L_StMd15_Rsp_Val/1
  MdXX_RspToNetWork_Cal_sys/9(IfVeSMSuHMI2L_StMd16_Rsp_Val_write) -> IfVeSMSuHMI2L_StMd16_Rsp_Val/1
  MdXX_RspToNetWork_Cal_sys/10(IfVeSMSuHMI2L_StMd17_Rsp_Val_write) -> IfVeSMSuHMI2L_StMd17_Rsp_Val/1
  MdXX_RspToNetWork_Cal_sys/11(IfVeSMSuHMI2L_StMd18_Rsp_Val_write) -> IfVeSMSuHMI2L_StMd18_Rsp_Val/1
  MdXX_RspToNetWork_Cal_sys/12(IfVeSMSuHMI2L_StMd19_Rsp_Val_write) -> IfVeSMSuHMI2L_StMd19_Rsp_Val/1
  MdXX_RspToNetWork_Cal_sys/13(IfVeSMSuHMI2L_StMd2_Rsp_Val_write) -> IfVeSMSuHMI2L_StMd2_Rsp_Val/1
  MdXX_RspToNetWork_Cal_sys/14(IfVeSMSuHMI2L_StMd20_Rsp_Val_write) -> IfVeSMSuHMI2L_StMd20_Rsp_Val/1
  MdXX_RspToNetWork_Cal_sys/15(IfVeSMSuHMI2L_StMd21_Rsp_Val_write) -> IfVeSMSuHMI2L_StMd21_Rsp_Val/1
  MdXX_RspToNetWork_Cal_sys/16(IfVeSMSuHMI2L_StMd22_Rsp_Val_write) -> IfVeSMSuHMI2L_StMd22_Rsp_Val/1
  MdXX_RspToNetWork_Cal_sys/17(IfVeSMSuHMI2L_StMd23_Rsp_Val_write) -> IfVeSMSuHMI2L_StMd23_Rsp_Val/1
  MdXX_RspToNetWork_Cal_sys/18(IfVeSMSuHMI2L_StMd24_Rsp_Val_write) -> IfVeSMSuHMI2L_StMd24_Rsp_Val/1
  MdXX_RspToNetWork_Cal_sys/19(IfVeSMSuHMI2L_StMd25_Rsp_Val_write) -> IfVeSMSuHMI2L_StMd25_Rsp_Val/1
  MdXX_RspToNetWork_Cal_sys/20(IfVeSMSuHMI2L_StMd26_Rsp_Val_write) -> IfVeSMSuHMI2L_StMd26_Rsp_Val/1
  MdXX_RspToNetWork_Cal_sys/21(IfVeSMSuHMI2L_StMd27_Rsp_Val_write) -> IfVeSMSuHMI2L_StMd27_Rsp_Val/1
  MdXX_RspToNetWork_Cal_sys/22(IfVeSMSuHMI2L_StMd28_Rsp_Val_write) -> IfVeSMSuHMI2L_StMd28_Rsp_Val/1
  MdXX_RspToNetWork_Cal_sys/23(IfVeSMSuHMI2L_StMd29_Rsp_Val_write) -> IfVeSMSuHMI2L_StMd29_Rsp_Val/1
  MdXX_RspToNetWork_Cal_sys/24(IfVeSMSuHMI2L_StMd3_Rsp_Val_write) -> IfVeSMSuHMI2L_StMd3_Rsp_Val/1
  MdXX_RspToNetWork_Cal_sys/25(IfVeSMSuHMI2L_StMd30_Rsp_Val_write) -> IfVeSMSuHMI2L_StMd30_Rsp_Val/1
  MdXX_RspToNetWork_Cal_sys/26(IfVeSMSuHMI2L_StMd31_Rsp_Val_write) -> IfVeSMSuHMI2L_StMd31_Rsp_Val/1
  MdXX_RspToNetWork_Cal_sys/27(IfVeSMSuHMI2L_StMd32_Rsp_Val_write) -> IfVeSMSuHMI2L_StMd32_Rsp_Val/1
  MdXX_RspToNetWork_Cal_sys/28(IfVeSMSuHMI2L_StMd4_Rsp_Val_write) -> IfVeSMSuHMI2L_StMd4_Rsp_Val/1
  MdXX_RspToNetWork_Cal_sys/29(IfVeSMSuHMI2L_StMd5_Rsp_Val_write) -> IfVeSMSuHMI2L_StMd5_Rsp_Val/1
  MdXX_RspToNetWork_Cal_sys/30(IfVeSMSuHMI2L_StMd6_Rsp_Val_write) -> IfVeSMSuHMI2L_StMd6_Rsp_Val/1
  MdXX_RspToNetWork_Cal_sys/31(IfVeSMSuHMI2L_StMd7_Rsp_Val_write) -> IfVeSMSuHMI2L_StMd7_Rsp_Val/1
  MdXX_RspToNetWork_Cal_sys/32(IfVeSMSuHMI2L_StMd8_Rsp_Val_write) -> IfVeSMSuHMI2L_StMd8_Rsp_Val/1
  MdXX_RspToNetWork_Cal_sys/33(IfVeSMSuHMI2L_StMd9_Rsp_Val_write) -> IfVeSMSuHMI2L_StMd9_Rsp_Val/1
  MdXX_RspToNetWork_Cal_sys/34(IfVeSMSuHMI2R_StMd1_Rsp_Val_write) -> IfVeSMSuHMI2R_StMd1_Rsp_Val/1
  MdXX_RspToNetWork_Cal_sys/35(IfVeSMSuHMI2R_StMd10_Rsp_Val_write) -> IfVeSMSuHMI2R_StMd10_Rsp_Val/1
  MdXX_RspToNetWork_Cal_sys/36(IfVeSMSuHMI2R_StMd11_Rsp_Val_write) -> IfVeSMSuHMI2R_StMd11_Rsp_Val/1
  MdXX_RspToNetWork_Cal_sys/37(IfVeSMSuHMI2R_StMd12_Rsp_Val_write) -> IfVeSMSuHMI2R_StMd12_Rsp_Val/1
  MdXX_RspToNetWork_Cal_sys/38(IfVeSMSuHMI2R_StMd13_Rsp_Val_write) -> IfVeSMSuHMI2R_StMd13_Rsp_Val/1
  MdXX_RspToNetWork_Cal_sys/39(IfVeSMSuHMI2R_StMd14_Rsp_Val_write) -> IfVeSMSuHMI2R_StMd14_Rsp_Val/1
  MdXX_RspToNetWork_Cal_sys/40(IfVeSMSuHMI2R_StMd15_Rsp_Val_write) -> IfVeSMSuHMI2R_StMd15_Rsp_Val/1
  MdXX_RspToNetWork_Cal_sys/41(IfVeSMSuHMI2R_StMd16_Rsp_Val_write) -> IfVeSMSuHMI2R_StMd16_Rsp_Val/1
  MdXX_RspToNetWork_Cal_sys/42(IfVeSMSuHMI2R_StMd17_Rsp_Val_write) -> IfVeSMSuHMI2R_StMd17_Rsp_Val/1
  MdXX_RspToNetWork_Cal_sys/43(IfVeSMSuHMI2R_StMd18_Rsp_Val_write) -> IfVeSMSuHMI2R_StMd18_Rsp_Val/1
  MdXX_RspToNetWork_Cal_sys/44(IfVeSMSuHMI2R_StMd19_Rsp_Val_write) -> IfVeSMSuHMI2R_StMd19_Rsp_Val/1
  MdXX_RspToNetWork_Cal_sys/45(IfVeSMSuHMI2R_StMd2_Rsp_Val_write) -> IfVeSMSuHMI2R_StMd2_Rsp_Val/1
  MdXX_RspToNetWork_Cal_sys/46(IfVeSMSuHMI2R_StMd20_Rsp_Val_write) -> IfVeSMSuHMI2R_StMd20_Rsp_Val/1
  MdXX_RspToNetWork_Cal_sys/47(IfVeSMSuHMI2R_StMd21_Rsp_Val_write) -> IfVeSMSuHMI2R_StMd21_Rsp_Val/1
  MdXX_RspToNetWork_Cal_sys/48(IfVeSMSuHMI2R_StMd22_Rsp_Val_write) -> IfVeSMSuHMI2R_StMd22_Rsp_Val/1
  MdXX_RspToNetWork_Cal_sys/49(IfVeSMSuHMI2R_StMd23_Rsp_Val_write) -> IfVeSMSuHMI2R_StMd23_Rsp_Val/1
  MdXX_RspToNetWork_Cal_sys/50(IfVeSMSuHMI2R_StMd24_Rsp_Val_write) -> IfVeSMSuHMI2R_StMd24_Rsp_Val/1
  MdXX_RspToNetWork_Cal_sys/51(IfVeSMSuHMI2R_StMd25_Rsp_Val_write) -> IfVeSMSuHMI2R_StMd25_Rsp_Val/1
  MdXX_RspToNetWork_Cal_sys/52(IfVeSMSuHMI2R_StMd26_Rsp_Val_write) -> IfVeSMSuHMI2R_StMd26_Rsp_Val/1
  MdXX_RspToNetWork_Cal_sys/53(IfVeSMSuHMI2R_StMd27_Rsp_Val_write) -> IfVeSMSuHMI2R_StMd27_Rsp_Val/1
  MdXX_RspToNetWork_Cal_sys/54(IfVeSMSuHMI2R_StMd28_Rsp_Val_write) -> IfVeSMSuHMI2R_StMd28_Rsp_Val/1
  MdXX_RspToNetWork_Cal_sys/55(IfVeSMSuHMI2R_StMd29_Rsp_Val_write) -> IfVeSMSuHMI2R_StMd29_Rsp_Val/1
  MdXX_RspToNetWork_Cal_sys/56(IfVeSMSuHMI2R_StMd3_Rsp_Val_write) -> IfVeSMSuHMI2R_StMd3_Rsp_Val/1
  MdXX_RspToNetWork_Cal_sys/57(IfVeSMSuHMI2R_StMd30_Rsp_Val_write) -> IfVeSMSuHMI2R_StMd30_Rsp_Val/1
  MdXX_RspToNetWork_Cal_sys/58(IfVeSMSuHMI2R_StMd31_Rsp_Val_write) -> IfVeSMSuHMI2R_StMd31_Rsp_Val/1
  MdXX_RspToNetWork_Cal_sys/59(IfVeSMSuHMI2R_StMd32_Rsp_Val_write) -> IfVeSMSuHMI2R_StMd32_Rsp_Val/1
  MdXX_RspToNetWork_Cal_sys/60(IfVeSMSuHMI2R_StMd4_Rsp_Val_write) -> IfVeSMSuHMI2R_StMd4_Rsp_Val/1
  MdXX_RspToNetWork_Cal_sys/61(IfVeSMSuHMI2R_StMd5_Rsp_Val_write) -> IfVeSMSuHMI2R_StMd5_Rsp_Val/1
  MdXX_RspToNetWork_Cal_sys/62(IfVeSMSuHMI2R_StMd6_Rsp_Val_write) -> IfVeSMSuHMI2R_StMd6_Rsp_Val/1
  MdXX_RspToNetWork_Cal_sys/63(IfVeSMSuHMI2R_StMd7_Rsp_Val_write) -> IfVeSMSuHMI2R_StMd7_Rsp_Val/1
  MdXX_RspToNetWork_Cal_sys/64(IfVeSMSuHMI2R_StMd8_Rsp_Val_write) -> IfVeSMSuHMI2R_StMd8_Rsp_Val/1
  MdXX_RspToNetWork_Cal_sys/65(IfVeSMSuHMI2R_StMd9_Rsp_Val_write) -> IfVeSMSuHMI2R_StMd9_Rsp_Val/1
  MdXX_RspToNetWork_Cal_sys/66(IfVeSMSuStPassCmprtMd10RclRspStat_Val_write) -> IfVeSMSuStPassCmprtMd10RclRspStat_Val/1
  MdXX_RspToNetWork_Cal_sys/67(IfVeSMSuStPassCmprtMd11RclRspStat_Val_write) -> IfVeSMSuStPassCmprtMd11RclRspStat_Val/1
  MdXX_RspToNetWork_Cal_sys/68(IfVeSMSuStPassCmprtMd12RclRspStat_Val_write) -> IfVeSMSuStPassCmprtMd12RclRspStat_Val/1
  MdXX_RspToNetWork_Cal_sys/69(IfVeSMSuStPassCmprtMd13RclRspStat_Val_write) -> IfVeSMSuStPassCmprtMd13RclRspStat_Val/1
  MdXX_RspToNetWork_Cal_sys/70(IfVeSMSuStPassCmprtMd14RclRspStat_Val_write) -> IfVeSMSuStPassCmprtMd14RclRspStat_Val/1
  MdXX_RspToNetWork_Cal_sys/71(IfVeSMSuStPassCmprtMd15RclRspStat_Val_write) -> IfVeSMSuStPassCmprtMd15RclRspStat_Val/1
  MdXX_RspToNetWork_Cal_sys/72(IfVeSMSuStPassCmprtMd16RclRspStat_Val_write) -> IfVeSMSuStPassCmprtMd16RclRspStat_Val/1
  MdXX_RspToNetWork_Cal_sys/73(IfVeSMSuStPassCmprtMd17RclRspStat_Val_write) -> IfVeSMSuStPassCmprtMd17RclRspStat_Val/1
  MdXX_RspToNetWork_Cal_sys/74(IfVeSMSuStPassCmprtMd18RclRspStat_Val_write) -> IfVeSMSuStPassCmprtMd18RclRspStat_Val/1
  MdXX_RspToNetWork_Cal_sys/75(IfVeSMSuStPassCmprtMd19RclRspStat_Val_write) -> IfVeSMSuStPassCmprtMd19RclRspStat_Val/1
  MdXX_RspToNetWork_Cal_sys/76(IfVeSMSuStPassCmprtMd1RclRspStat_Val_write) -> IfVeSMSuStPassCmprtMd1RclRspStat_Val/1
  MdXX_RspToNetWork_Cal_sys/77(IfVeSMSuStPassCmprtMd20RclRspStat_Val_write) -> IfVeSMSuStPassCmprtMd20RclRspStat_Val/1
  MdXX_RspToNetWork_Cal_sys/78(IfVeSMSuStPassCmprtMd21RclRspStat_Val_write) -> IfVeSMSuStPassCmprtMd21RclRspStat_Val/1
  MdXX_RspToNetWork_Cal_sys/79(IfVeSMSuStPassCmprtMd22RclRspStat_Val_write) -> IfVeSMSuStPassCmprtMd22RclRspStat_Val/1
  MdXX_RspToNetWork_Cal_sys/80(IfVeSMSuStPassCmprtMd23RclRspStat_Val_write) -> IfVeSMSuStPassCmprtMd23RclRspStat_Val/1
  MdXX_RspToNetWork_Cal_sys/81(IfVeSMSuStPassCmprtMd24RclRspStat_Val_write) -> IfVeSMSuStPassCmprtMd24RclRspStat_Val/1
  MdXX_RspToNetWork_Cal_sys/82(IfVeSMSuStPassCmprtMd25RclRspStat_Val_write) -> IfVeSMSuStPassCmprtMd25RclRspStat_Val/1
  MdXX_RspToNetWork_Cal_sys/83(IfVeSMSuStPassCmprtMd26RclRspStat_Val_write) -> IfVeSMSuStPassCmprtMd26RclRspStat_Val/1
  MdXX_RspToNetWork_Cal_sys/84(IfVeSMSuStPassCmprtMd27RclRspStat_Val_write) -> IfVeSMSuStPassCmprtMd27RclRspStat_Val/1
  MdXX_RspToNetWork_Cal_sys/85(IfVeSMSuStPassCmprtMd28RclRspStat_Val_write) -> IfVeSMSuStPassCmprtMd28RclRspStat_Val/1
  MdXX_RspToNetWork_Cal_sys/86(IfVeSMSuStPassCmprtMd29RclRspStat_Val_write) -> IfVeSMSuStPassCmprtMd29RclRspStat_Val/1
  MdXX_RspToNetWork_Cal_sys/87(IfVeSMSuStPassCmprtMd2RclRspStat_Val_write) -> IfVeSMSuStPassCmprtMd2RclRspStat_Val/1
  MdXX_RspToNetWork_Cal_sys/88(IfVeSMSuStPassCmprtMd30RclRspStat_Val_write) -> IfVeSMSuStPassCmprtMd30RclRspStat_Val/1
  MdXX_RspToNetWork_Cal_sys/89(IfVeSMSuStPassCmprtMd31RclRspStat_Val_write) -> IfVeSMSuStPassCmprtMd31RclRspStat_Val/1
  MdXX_RspToNetWork_Cal_sys/90(IfVeSMSuStPassCmprtMd32RclRspStat_Val_write) -> IfVeSMSuStPassCmprtMd32RclRspStat_Val/1
  MdXX_RspToNetWork_Cal_sys/91(IfVeSMSuStPassCmprtMd3RclRspStat_Val_write) -> IfVeSMSuStPassCmprtMd3RclRspStat_Val/1
  MdXX_RspToNetWork_Cal_sys/92(IfVeSMSuStPassCmprtMd4RclRspStat_Val_write) -> IfVeSMSuStPassCmprtMd4RclRspStat_Val/1
  MdXX_RspToNetWork_Cal_sys/93(IfVeSMSuStPassCmprtMd5RclRspStat_Val_write) -> IfVeSMSuStPassCmprtMd5RclRspStat_Val/1
  MdXX_RspToNetWork_Cal_sys/94(IfVeSMSuStPassCmprtMd6RclRspStat_Val_write) -> IfVeSMSuStPassCmprtMd6RclRspStat_Val/1
  MdXX_RspToNetWork_Cal_sys/95(IfVeSMSuStPassCmprtMd7RclRspStat_Val_write) -> IfVeSMSuStPassCmprtMd7RclRspStat_Val/1
  MdXX_RspToNetWork_Cal_sys/96(IfVeSMSuStPassCmprtMd8RclRspStat_Val_write) -> IfVeSMSuStPassCmprtMd8RclRspStat_Val/1
  MdXX_RspToNetWork_Cal_sys/97(IfVeSMSuStPassCmprtMd9RclRspStat_Val_write) -> IfVeSMSuStPassCmprtMd9RclRspStat_Val/1
  MdXX_RspToNetWork_Cal_sys/98(IfVeSMSuStSrv_StMd1_Rsp_Val_write) -> IfVeSMSuStSrv_StMd1_Rsp_Val/1
  MdXX_RspToNetWork_Cal_sys/99(IfVeSMSuStSrv_StMd10_Rsp_Val_write) -> IfVeSMSuStSrv_StMd10_Rsp_Val/1
  MdXX_RspToNetWork_Cal_sys/100(IfVeSMSuStSrv_StMd11_Rsp_Val_write) -> IfVeSMSuStSrv_StMd11_Rsp_Val/1
  MdXX_RspToNetWork_Cal_sys/101(IfVeSMSuStSrv_StMd12_Rsp_Val_write) -> IfVeSMSuStSrv_StMd12_Rsp_Val/1
  MdXX_RspToNetWork_Cal_sys/102(IfVeSMSuStSrv_StMd13_Rsp_Val_write) -> IfVeSMSuStSrv_StMd13_Rsp_Val/1
  MdXX_RspToNetWork_Cal_sys/103(IfVeSMSuStSrv_StMd14_Rsp_Val_write) -> IfVeSMSuStSrv_StMd14_Rsp_Val/1
  MdXX_RspToNetWork_Cal_sys/104(IfVeSMSuStSrv_StMd15_Rsp_Val_write) -> IfVeSMSuStSrv_StMd15_Rsp_Val/1
  MdXX_RspToNetWork_Cal_sys/105(IfVeSMSuStSrv_StMd16_Rsp_Val_write) -> IfVeSMSuStSrv_StMd16_Rsp_Val/1
  MdXX_RspToNetWork_Cal_sys/106(IfVeSMSuStSrv_StMd17_Rsp_Val_write) -> IfVeSMSuStSrv_StMd17_Rsp_Val/1
  MdXX_RspToNetWork_Cal_sys/107(IfVeSMSuStSrv_StMd18_Rsp_Val_write) -> IfVeSMSuStSrv_StMd18_Rsp_Val/1
  MdXX_RspToNetWork_Cal_sys/108(IfVeSMSuStSrv_StMd19_Rsp_Val_write) -> IfVeSMSuStSrv_StMd19_Rsp_Val/1
  MdXX_RspToNetWork_Cal_sys/109(IfVeSMSuStSrv_StMd2_Rsp_Val_write) -> IfVeSMSuStSrv_StMd2_Rsp_Val/1
  MdXX_RspToNetWork_Cal_sys/110(IfVeSMSuStSrv_StMd20_Rsp_Val_write) -> IfVeSMSuStSrv_StMd20_Rsp_Val/1
  MdXX_RspToNetWork_Cal_sys/111(IfVeSMSuStSrv_StMd21_Rsp_Val_write) -> IfVeSMSuStSrv_StMd21_Rsp_Val/1
  MdXX_RspToNetWork_Cal_sys/112(IfVeSMSuStSrv_StMd22_Rsp_Val_write) -> IfVeSMSuStSrv_StMd22_Rsp_Val/1
  MdXX_RspToNetWork_Cal_sys/113(IfVeSMSuStSrv_StMd23_Rsp_Val_write) -> IfVeSMSuStSrv_StMd23_Rsp_Val/1
  MdXX_RspToNetWork_Cal_sys/114(IfVeSMSuStSrv_StMd24_Rsp_Val_write) -> IfVeSMSuStSrv_StMd24_Rsp_Val/1
  MdXX_RspToNetWork_Cal_sys/115(IfVeSMSuStSrv_StMd25_Rsp_Val_write) -> IfVeSMSuStSrv_StMd25_Rsp_Val/1
  MdXX_RspToNetWork_Cal_sys/116(IfVeSMSuStSrv_StMd26_Rsp_Val_write) -> IfVeSMSuStSrv_StMd26_Rsp_Val/1
  MdXX_RspToNetWork_Cal_sys/117(IfVeSMSuStSrv_StMd27_Rsp_Val_write) -> IfVeSMSuStSrv_StMd27_Rsp_Val/1
  MdXX_RspToNetWork_Cal_sys/118(IfVeSMSuStSrv_StMd28_Rsp_Val_write) -> IfVeSMSuStSrv_StMd28_Rsp_Val/1
  MdXX_RspToNetWork_Cal_sys/119(IfVeSMSuStSrv_StMd29_Rsp_Val_write) -> IfVeSMSuStSrv_StMd29_Rsp_Val/1
  MdXX_RspToNetWork_Cal_sys/120(IfVeSMSuStSrv_StMd3_Rsp_Val_write) -> IfVeSMSuStSrv_StMd3_Rsp_Val/1
  MdXX_RspToNetWork_Cal_sys/121(IfVeSMSuStSrv_StMd30_Rsp_Val_write) -> IfVeSMSuStSrv_StMd30_Rsp_Val/1
  MdXX_RspToNetWork_Cal_sys/122(IfVeSMSuStSrv_StMd31_Rsp_Val_write) -> IfVeSMSuStSrv_StMd31_Rsp_Val/1
  MdXX_RspToNetWork_Cal_sys/123(IfVeSMSuStSrv_StMd32_Rsp_Val_write) -> IfVeSMSuStSrv_StMd32_Rsp_Val/1
  MdXX_RspToNetWork_Cal_sys/124(IfVeSMSuStSrv_StMd4_Rsp_Val_write) -> IfVeSMSuStSrv_StMd4_Rsp_Val/1
  MdXX_RspToNetWork_Cal_sys/125(IfVeSMSuStSrv_StMd5_Rsp_Val_write) -> IfVeSMSuStSrv_StMd5_Rsp_Val/1
  MdXX_RspToNetWork_Cal_sys/126(IfVeSMSuStSrv_StMd6_Rsp_Val_write) -> IfVeSMSuStSrv_StMd6_Rsp_Val/1
  MdXX_RspToNetWork_Cal_sys/127(IfVeSMSuStSrv_StMd7_Rsp_Val_write) -> IfVeSMSuStSrv_StMd7_Rsp_Val/1
  MdXX_RspToNetWork_Cal_sys/128(IfVeSMSuStSrv_StMd8_Rsp_Val_write) -> IfVeSMSuStSrv_StMd8_Rsp_Val/1
  MdXX_RspToNetWork_Cal_sys/129(IfVeSMSuStSrv_StMd9_Rsp_Val_write) -> IfVeSMSuStSrv_StMd9_Rsp_Val/1
  MdXX_RspToNetWork_Cal_sys/130(IfVeSMSuStPassCmprtMd53RclRspStat_Val_write) -> IfVeSMSuStPassCmprtMd53RclRspStat_Val/1
  MdXX_RspToNetWork_Cal_sys/131(IfVeSMSuStPassCmprtMd56RclRspStat_Val_write) -> IfVeSMSuStPassCmprtMd56RclRspStat_Val/1
  MdXX_RspToNetWork_Cal_sys/132(IfVeSMSuStSrv_StMd53_Rsp_Val_write) -> IfVeSMSuStSrv_StMd53_Rsp_Val/1
  MdXX_RspToNetWork_Cal_sys/133(IfVeSMSuStSrv_StMd56_Rsp_Val_write) -> IfVeSMSuStSrv_StMd56_Rsp_Val/1
  MdXX_RspToNetWork_Cal_sys/134(IfVeSMSuStPassCmprtMd57RclRspStat_Val_write) -> IfVeSMSuStPassCmprtMd57RclRspStat_Val/1
  MdXX_RspToNetWork_Cal_sys/135(IfVeSMSuStPassCmprtMd58RclRspStat_Val_write) -> IfVeSMSuStPassCmprtMd58RclRspStat_Val/1
  MdXX_RspToNetWork_Cal_sys/136(IfVeSMSuStPassCmprtMd61RclRspStat_Val_write) -> IfVeSMSuStPassCmprtMd61RclRspStat_Val/1
  MdXX_RspToNetWork_Cal_sys/137(IfVeSMSuStPassCmprtMd62RclRspStat_Val_write) -> IfVeSMSuStPassCmprtMd62RclRspStat_Val/1
